simulink library "ECEFtoJ2000"  (R2014b)
settings: Solver=ode45  StartTime=0.0  StopTime=10.0  RelTol=1e-3
undefined symbols (not defined in the file or in its folder): ConfParam
settings Model: Creator=Hp  LastModifiedBy=Hp

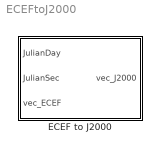
== system ECEFtoJ2000 ==
  ECEF to J2000 : Subsystem

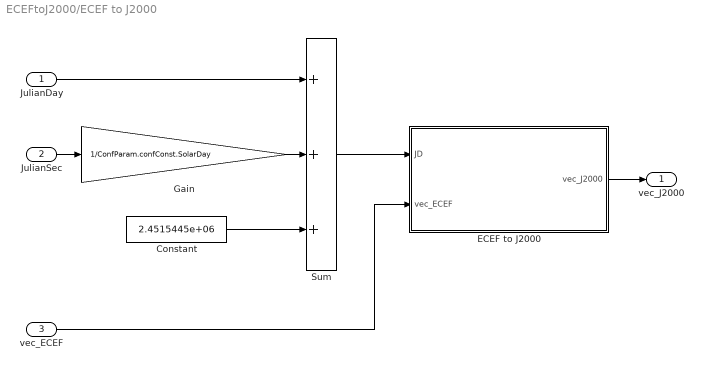
== system ECEFtoJ2000/ECEF to J2000 ==
  JulianDay : Inport
  JulianSec : Inport  Port=2
  vec_ECEF : Inport  Port=3
  Constant : Constant  Value=2.4515445e+06
  ECEF to J2000 : MATLAB Function  TreatAsAtomicUnit=on
  Gain : Gain  Gain=1/ConfParam.confConst.SolarDay
  Sum : Sum  Inputs=+++
  vec_J2000 : Outport
  wires:
  vec_ECEF/1 -> ECEF to J2000/2(vec_ECEF)
  ECEF to J2000/1(vec_J2000) -> vec_J2000/1
  Constant/1 -> Sum/3
  JulianSec/1 -> Gain/1
  JulianDay/1 -> Sum/1
  Gain/1 -> Sum/2
  Sum/1 -> ECEF to J2000/1(JD)

== matlab function ECEFtoJ2000/ECEF to J2000/ECEF to J2000 ==
  data: JD input; vec_J2000 output; vec_ECEF input
function vec_J2000 = ECEFtoJ2000(JD, vec_ECEF)

%Calculate the Greenwich Apparent Sideral Time (THETA)
%See http://www.cdeagle.com/omnum/pdf/csystems.pdf equation 27
THETA = JD2GAST(JD);

%Assemble the transformation matricies to go from ECEF to ECI
%See http://www.cdeagle.com/omnum/pdf/csystems.pdf equation 26
vec_J2000 = squeeze(MultiDimMatrixMultiply(MultiDimMatrixTranspose(T3D(THETA)),vec_ECEF));
%----------------------------- End Code-----------------------------------%
end
